simulink model "rti1401_program_nova"  (R2017b)
settings: Solver=ode1  StartTime=0.0  StopTime=Inf  FixedStep=0.001  RelTol=1e-3  EnableMultiTasking=on
PreLoadFcn:
  | dataCar
  | load_vars
  | structAero
  | structEstimPar
  | structSensors
  | structSettings
PostLoadFcn:
  | , if any(exist('dsrtsu_mdlpostloadfcn', 'file') == [2, 3, 6]), try dsrtsu_mdlpostloadfcn('Execute', bdroot); catch fprintf('Error in PostLoadFcn (dsrtsu_mdlpostloadfcn) for model "%s":\n %s\n', bdroot, lasterr); end, end,
InitFcn:
  | dataCar
  | load_vars
  | structAero
  | structEstimPar
  | structSensors
  | structSettings
StartFcn:
  | dataCar
  | load_vars
  | structAero
  | structEstimPar
  | structSensors
  | structSettings
values from neighbouring files (symbols this model uses):
  Throttle_limits = [0.15, 0.90, 0.16, 0.92]    [load_vars.m]
libraries: rtican x44, hdlsllib x32, simulink x8, rti1401lib_II_base x1, fuzblock x1
(part 3 of 11)

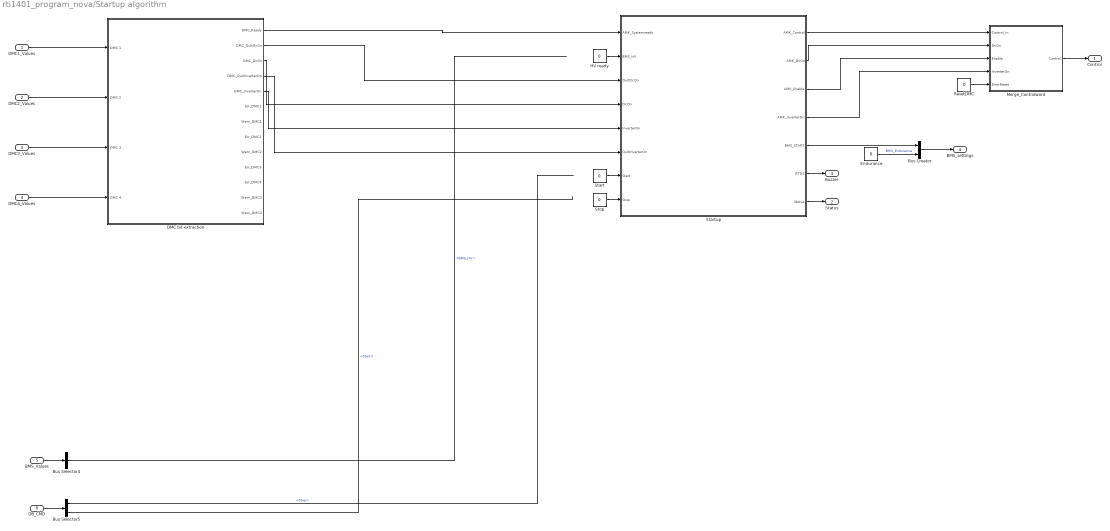
== system rti1401_program_nova/Startup algorithm ==
  DMC1_Values : Inport
  DMC2_Values : Inport  Port=2
  DMC3_Values : Inport  Port=3
  DMC4_Values : Inport  Port=4
  BMS_Values : Inport  Port=5
  DB_CMD : Inport  Port=6
  Bus Creator : BusCreator  Inputs=2
  Bus Selector4 : BusSelector  OutputSignals=BMS_HV
  Bus Selector5 : BusSelector  OutputSignals=Stop,Start
  DMC bit extraction : Subsystem
  Endurance : Constant  Value=0
  HV ready : Constant  Value=0
  Merge_Controlword : Subsystem
  ResetDMC : Constant  Value=0
  Start : Constant  Value=0
  Startup : Stateflow chart  TreatAsAtomicUnit=on
  Stop : Constant  Value=0
  Control : Outport
  Status : Outport  Port=2
  Buzzer : Outport  Port=3
  BMS_settings : Outport  Port=4
  wires:
  DB_CMD/1 -> Bus Selector5/1
  BMS_Values/1 -> Bus Selector4/1
  DMC1_Values/1 -> DMC bit extraction/1(DMC 1)
  DMC2_Values/1 -> DMC bit extraction/2(DMC 2)
  DMC3_Values/1 -> DMC bit extraction/3(DMC 3)
  DMC4_Values/1 -> DMC bit extraction/4(DMC 4)
  DMC bit extraction/1(DMC_Ready) -> Startup/1(AMK_Systemready)
  Bus Selector5/1 -> ?  "<Stop>"
  Bus Selector5/2 -> ?  "<Start>"
  Bus Selector4/1 -> ?  "<BMS_HV>"
  Startup/1(AMK_Control) -> Merge_Controlword/1(Control_in)
  Startup/2(AMK_DcOn) -> Merge_Controlword/2(DcOn)
  Startup/3(AMK_Enable) -> Merge_Controlword/3(Enable)
  Startup/4(AMK_InverterOn) -> Merge_Controlword/4(InverterOn)
  ResetDMC/1 -> Merge_Controlword/5(ErrorReset)
  Merge_Controlword/1(Control) -> Control/1
  Startup/7(Status) -> Status/1
  Startup/6(RTDS) -> Buzzer/1
  Startup/5(BMS_START) -> Bus Creator/1
  Endurance/1 -> Bus Creator/2  "BMS_Endurance"
  Bus Creator/1 -> BMS_settings/1
  HV ready/1 -> Startup/2(BMS_HV)
  DMC bit extraction/2(DMC_QuitDcOn) -> Startup/3(QuitDcOn)
  DMC bit extraction/3(DMC_DcOn) -> Startup/4(DcOn)
  DMC bit extraction/5(DMC_InverterOn) -> Startup/5(InverterOn)
  DMC bit extraction/4(DMC_QuitInverterOn) -> Startup/6(QuitInverterOn)
  Start/1 -> Startup/7(Start)
  Stop/1 -> Startup/8(Stop)

== system rti1401_program_nova/Inputs/Batpack ==
  Bus Creator : BusCreator  Inputs=19
  CAN_BMS_Values : rtican/RTICAN Receive (RX)   Reserved1=[]  Reserved2=[]  Reserved3=[]  Reserved4=[]  SfcnMessage=[]  Msg_Struct=[]  BoardTypeNo=[]  BoardNo=[]  ChannelNo=[]  Parameters=[]  DialogFcn=[]  UnitName=[]  Revision=[]  UnitValues=[]  DSProperties=struct('RTI',struct('Version',uint32(5),'BlockType',struct('isSLSource',uint8(1),'isSLSink',uint8(1),'isHWSource',uint8(0),'isHWSink',uint8(0),'isSetup',uint8(0),'isInline',uint8(1),'isNonInline',uint8(0),'isInterrupt',uint8(0),'isChannelwise',uint8(0)),'IOBoardType','RTICAN','UnitType','MESSAGE','Identifier','RX','DialogType','MSVC','BlockSet','RTICAN','SlaveProcessor','CAN'))  RTIBlockInterface=struct('OutputPortsWidth',int32([1 1 1 1 1 1 1 1 1 1 1 1 1 1 1 1 1 1 1]),'OutputPortsActive',[1 1 1 1 1 1 1 1 1 1 1 1 1 1 1 1 1 1 1],'OutputPortsName',{{'BMS_Total_Voltage','BMS_SoC','BMS_M1','BMS_M2','BMS_M3','BMS_M4','BMS_BOTS','BMS_Inertia','BMS_Interlock','BMS_BSPD','BMS_TSMS','BMS_IMD','BMS_Status','BMS_Voltage_Err','BMS_Temp_Err','BMS_HVD','BMS_Temp_Warn','BMS_Voltage_Warn','BMS_HV'}},'OutputPortsDataType',{{'SS_UINT16','SS_UINT16','SS_BOOLEAN','SS_BOOLEAN','SS_BOOLEAN','SS_BOOLEAN','SS_BOOLEAN','SS_BOOLEAN','SS_BOOLEAN','SS_BOOLEAN','SS_BOOLEAN','SS_BOOLEAN','SS_BOOLEAN','SS_BOOLEAN','SS_BOOLEAN','SS_BOOLEAN','SS_BOOLEAN','SS_BOOLEAN','SS_BOOLEAN'}},'OutputPortsLabel',{{'BMS_Total_Voltage','BMS_SoC','BMS_M1','BMS_M2','BMS_M3','BMS_M4','BMS_BOTS','BMS_Inertia','BMS_Interlock','BMS_BSPD','BMS_TSMS','BMS_IMD','BMS_Status','BMS_Voltage_Err','BMS_Temp_Err','BMS_HVD','BMS_Temp_Warn','BMS_Voltage_Warn','BMS_HV'}},'OutputPortsLabelMode','ON','InputPortsWidth',int32(0),'InputPortsActive',0,'DialogFcn','rtican_message_interface_gui','BlockDisplay',{{'','center'}},'IconTransparency','on','ParameterTunableNames',{{}},'InitLevel',3,'BlockName',struct('Token',{{'CAN_TYPE','_RX_M','_C'}},'BlockParam',{{'BoardTypeNo','BoardNo','ChannelNo'}}),'SampleTime',{{-1}},'TriggerPort',{{'none'}},'EnablePort',{{'none'}})  RTIBlockParameters=struct('BoardTypeNo',{{1,'OFF',[]}},'BoardNo',{{2,'ON',[1 16]}},'ChannelNo',{{2,'ON',[1 2]}},'Parameters',{{struct('DataFileSupport',struct('DataFileSelectedMaster',0,'DataFileSelectedLocal',0,'DataFileName',['<no datafile support>|'],'DataFileDate','','SelectedFile',['<no file selected>']),'Options',struct('StatusSelected',0,'TimeSelected',0,'DeltaTimeSelected',0,'BytePortSelected',0,'MessageLengthSelected',0,'TriggerPort',struct('Selected',0,'TriggerType',0),'UserCoding',struct('Selected',0,'InterfaceFile','UserDecodingFile','FcnName','UserDecodeFcn','InportSelected',0,'InportWidth',1,'OutportSelected',0,'OutportWidth',1),'EnablePortSelected',0,'SignalOnPortnameSelected',1,'UseRXService',0),'Message',struct('MsgOnBlocknameSelected',0,'MsgName','BMS_Values','MsgIdFormat',0,'MsgId',1,'MsgLength',7,'NumSignals',19,'SampleTime',-1,'Signal',struct('SgnName',{'BMS_Total_Voltage','BMS_SoC','BMS_M1','BMS_M2','BMS_M3','BMS_M4','BMS_BOTS','BMS_Inertia','BMS_Interlock','BMS_BSPD','BMS_TSMS','BMS_IMD','BMS_Status','BMS_Voltage_Err','BMS_Temp_Err','BMS_HVD','BMS_Temp_Warn','BMS_Voltage_Warn','BMS_HV'},'SgnStartBit',{0,16,32,33,34,35,36,37,38,39,40,41,42,43,44,45,46,47,48},'SgnLength',{16,16,1,1,1,1,1,1,1,1,1,1,1,1,1,1,1,1,1},'SgnType',{0,0,0,0,0,0,0,0,0,0,0,0,0,0,0,0,0,0,0},'ModeValue',{-1,-1,-1,-1,-1,-1,-1,-1,-1,-1,-1,-1,-1,-1,-1,-1,-1,-1,-1},'DataType',{0,0,0,0,0,0,0,0,0,0,0,0,0,0,0,0,0,0,0},'ByteLayout',{0,0,0,0,0,0,0,0,0,0,0,0,0,0,0,0,0,0,0},'Factor',{1,1,1,1,1,1,1,1,1,1,1,1,1,1,1,1,1,1,1},'Offset',{0,0,0,0,0,0,0,0,0,0,0,0,0,0,0,0,0,0,0},'SgnComment',{{''},{''},{''},{''},{''},{''},{''},{''},{''},{''},{''},{''},{''},{''},{''},{''},{''},{''},{''}},'SgnUnit',{'','','','','','','','','','','','','','','','','','',''},'Min',{0,0,0,0,0,0,0,0,0,0,0,0,0,0,0,0,0,0,0},'Max',{255,255,255,255,255,255,255,255,255,255,255,255,255,255,255,255,255,255,255},'SLDataType',{'SS_UINT16','SS_UINT16','SS_BOOLEAN','SS_BOOLEAN','SS_BOOLEAN','SS_BOOLEAN','SS_BOOLEAN','SS_BOOLEAN','SS_BOOLEAN','SS_BOOLEAN','SS_BOOLEAN','SS_BOOLEAN','SS_BOOLEAN','SS_BOOLEAN','SS_BOOLEAN','SS_BOOLEAN','SS_BOOLEAN','SS_BOOLEAN','SS_BOOLEAN'}),'MsgIdNumFormat',1,'MsgComment',{{''}}),'Version',1.2,'general',struct('isFromLib',0)),'OFF',[]}},'GroupId',{{struct('Group',{{'RTICAN'}},'No',4,'Behavior',{{'NAMECHANGE'}},'BlockType',{{'SINK'}},'NameChangeFlag',0),'OFF',[]}},'SFcnRTICANMessage',{{struct('MsgType','RX','SFcnPortType','Scalar','MsgName','BMS_Values','MsgIdFormat','STD','MsgId',1,'MsgLength',7,'NumSignals',19,'SampleTime',-1,'Signal',struct('SgnName',{'BMS_Total_Voltage','BMS_SoC','BMS_M1','BMS_M2','BMS_M3','BMS_M4','BMS_BOTS','BMS_Inertia','BMS_Interlock','BMS_BSPD','BMS_TSMS','BMS_IMD','BMS_Status','BMS_Voltage_Err','BMS_Temp_Err','BMS_HVD','BMS_Temp_Warn','BMS_Voltage_Warn','BMS_HV'},'SgnStartBit',{0,16,32,33,34,35,36,37,38,39,40,41,42,43,44,45,46,47,48},'SgnLength',{16,16,1,1,1,1,1,1,1,1,1,1,1,1,1,1,1,1,1},'SgnType',{'standard','standard','standard','standard','standard','standard','standard','standard','standard','standard','standard','standard','standard','standard','standard','standard','standard','standard','standard'},'ModeValue',{-1,-1,-1,-1,-1,-1,-1,-1,-1,-1,-1,-1,-1,-1,-1,-1,-1,-1,-1},'DataType',{['unsigned int'],['unsigned int'],['unsigned int'],['unsigned int'],['unsigned int'],['unsigned int'],['unsigned int'],['unsigned int'],['unsigned int'],['unsigned int'],['unsigned int'],['unsigned int'],['unsigned int'],['unsigned int'],['unsigned int'],['unsigned int'],['unsigned int'],['unsigned int'],['unsigned int']},'ByteLayout',{['little endian'],['little endian'],['little endian'],['little endian'],['little endian'],['little endian'],['little endian'],['little endian'],['little endian'],['little endian'],['little endian'],['little endian'],['little endian'],['little endian'],['little endian'],['little endian'],['little endian'],['little endian'],['little endian']},'Factor',{1,1,1,1,1,1,1,1,1,1,1,1,1,1,1,1,1,1,1},'Offset',{0,0,0,0,0,0,0,0,0,0,0,0,0,0,0,0,0,0,0},'SLDataType',{'SS_UINT16','SS_UINT16','SS_BOOLEAN','SS_BOOLEAN','SS_BOOLEAN','SS_BOOLEAN','SS_BOOLEAN','SS_BOOLEAN','SS_BOOLEAN','SS_BOOLEAN','SS_BOOLEAN','SS_BOOLEAN','SS_BOOLEAN','SS_BOOLEAN','SS_BOOLEAN','SS_BOOLEAN','SS_BOOLEAN','SS_BOOLEAN','SS_BOOLEAN'}),'StatusSelected','no','TimeSelected','no','DeltaTimeSelected','no','BytePortSelected','no','MessageLengthSelected','no','TriggerPort',struct('Selected','no','TriggerType',0),'UserCoding',struct('Selected','no','InterfaceFile','UserDecodingFile','FcnName','UserDecodeFcn','InportSelected','no','InportWidth',1,'OutportSelected','no','OutportWidth',1),'EnablePortSelected','no','UseRXService','no','BoardType','DS1','BoardNo',2,'ControllerNo',2),'OFF',[]}},'TLCFileName',{{'rtican_rx_message','OFF',[]}})  RTISFcnParameters=struct('SFcnRTICANMessage','struct','TLCFileName','char')  RTIBlockParaDefault=struct('BoardTypeNo',4302,'BoardNo',1,'ChannelNo',1,'Parameters',struct('DataFileSupport',struct('DataFileSelectedMaster',0,'DataFileSelectedLocal',0,'DataFileName','','DataFileDate','','SelectedFile',['<no file selected>']),'Options',struct('StatusSelected',1,'TimeSelected',1,'DeltaTimeSelected',1,'BytePortSelected',0,'MessageLengthSelected',0,'TriggerPort',struct('Selected',0,'TriggerType','rising'),'UserCoding',struct('Selected',0,'InterfaceFile','UserDecodingFile','FcnName','UserDecodeFcn','InportSelected',0,'InportWidth',1,'OutportSelected',0,'OutportWidth',1),'EnablePortSelected',0,'SignalOnPortnameSelected',1,'UseRXService',0),'Message',struct('MsgOnBlocknameSelected',0,'MsgName',['RX Message'],'MsgIdFormat',0,'MsgId',100,'MsgLength',8,'NumSignals',1,'SampleTime',-1,'Signal',struct('SgnName',['RX signal'],'SgnStartBit',0,'SgnLength',8,'SgnType',0,'ModeValue',-1,'DataType',0,'SLDataType','SS_DOUBLE','ByteLayout',0,'Factor',1,'Offset',0,'Min',0,'Max',255,'SgnComment',{{}},'SgnUnit',''),'MsgIdNumFormat',0,'MsgComment',{{''}}),'Version',1.2,'general',struct('isFromLib',1)),'GroupId',struct('Group',{{'RTICAN'}},'No',1,'Behavior',{{'NAMECHANGE'}},'BlockType',{{'SINK'}},'NameChangeFlag',0),'SFcnRTICANMessage',struct('MsgType','RX','MsgName',['RX Message'],'MsgIdFormat','STD','MsgId',100,'MsgLength',8,'NumSignals',1,'SampleTime',-1,'Signal',struct('SgnName',['RX signal'],'SgnStartBit',0,'SgnLength',8,'SgnType','standard','ModeValue',-1,'DataType',['unsigned int'],'ByteLayout',['little endian'],'SLDataType','SS_DOUBLE','Factor',1,'Offset',0),'StatusSelected','yes','TimeSelected','yes','DeltaTimeSelected','yes','BytePortSelected','no','MessageLengthSelected','no','EnablePortSelected','no','UserCoding',struct('Selected','no','InterfaceFile','UserDecodingFile','FcnName','UserDecodeFcn','InportSelected','no','InportWidth',1,'OutportSelected','no','OutportWidth',1),'TriggerPort',struct('Selected','no','TriggerType','rising'),'UseRXService','no','BoardType','DS4302','BoardNo',1,'ControllerNo',1,'SFcnPortType','Scalar'),'TLCFileName','rtican_rx_message')
      settings: AttributesFormatString=Group Id: RTICAN4\n
  BMS_Values : Outport
  wires:
  CAN_BMS_Values/19 -> Bus Creator/19  "BMS_HV"
  CAN_BMS_Values/18 -> Bus Creator/18  "BMS_Voltage_Warn"
  CAN_BMS_Values/17 -> Bus Creator/17  "BMS_Temp_Warn"
  CAN_BMS_Values/16 -> Bus Creator/16  "BMS_HVD"
  CAN_BMS_Values/15 -> Bus Creator/15  "BMS_Temp_Err"
  CAN_BMS_Values/14 -> Bus Creator/14  "BMS_Voltage_Err"
  CAN_BMS_Values/13 -> Bus Creator/13  "BMS_Status"
  CAN_BMS_Values/12 -> Bus Creator/12  "BMS_IMD"
  CAN_BMS_Values/11 -> Bus Creator/11  "BMS_TSMS"
  CAN_BMS_Values/10 -> Bus Creator/10  "BMS_BSPD"
  CAN_BMS_Values/9 -> Bus Creator/9  "BMS_Interlock"
  CAN_BMS_Values/8 -> Bus Creator/8  "BMS_Inertia"
  CAN_BMS_Values/7 -> Bus Creator/7  "BMS_BOTS"
  CAN_BMS_Values/6 -> Bus Creator/6  "BMS_M4"
  CAN_BMS_Values/5 -> Bus Creator/5  "BMS_M3"
  CAN_BMS_Values/4 -> Bus Creator/4  "BMS_M2"
  CAN_BMS_Values/3 -> Bus Creator/3  "BMS_M1"
  CAN_BMS_Values/2 -> Bus Creator/2  "BMS_SoC"
  CAN_BMS_Values/1 -> Bus Creator/1  "BMS_Total_Voltage"
  Bus Creator/1 -> BMS_Values/1

== system rti1401_program_nova/Inputs/Commands ==
  Bus Creator : BusCreator  Inputs=10
  CAN_TYPE1_RX_M1_C1 : rtican/RTICAN Receive (RX)   Reserved1=[]  Reserved2=[]  Reserved3=[]  Reserved4=[]  SfcnMessage=[]  Msg_Struct=[]  BoardTypeNo=[]  BoardNo=[]  ChannelNo=[]  Parameters=[]  DialogFcn=[]  UnitName=[]  Revision=[]  UnitValues=[]  DSProperties=struct('RTI',struct('Version',uint32(5),'BlockType',struct('isSLSource',uint8(1),'isSLSink',uint8(1),'isHWSource',uint8(0),'isHWSink',uint8(0),'isSetup',uint8(0),'isInline',uint8(1),'isNonInline',uint8(0),'isInterrupt',uint8(0),'isChannelwise',uint8(0)),'IOBoardType','RTICAN','UnitType','MESSAGE','Identifier','RX','DialogType','MSVC','BlockSet','RTICAN','SlaveProcessor','CAN'))  RTIBlockInterface=struct('OutputPortsWidth',int32([1 1 1 1 1 1 1 1 1]),'OutputPortsActive',[1 1 1 1 1 1 1 1 1],'OutputPortsName',{{'Start','Stop','TV','Power','MxFz','Regen','Traction','FxInf','YRC'}},'OutputPortsDataType',{{'SS_BOOLEAN','SS_BOOLEAN','SS_UINT8','SS_UINT8','SS_UINT8','SS_UINT8','SS_BOOLEAN','SS_BOOLEAN','SS_BOOLEAN'}},'OutputPortsLabel',{{'Start','Stop','TV','Power','MxFz','Regen','Traction','FxInf','YRC'}},'OutputPortsLabelMode','ON','InputPortsWidth',int32(0),'InputPortsActive',0,'DialogFcn','rtican_message_interface_gui','BlockDisplay',{{'','center'}},'IconTransparency','on','ParameterTunableNames',{{}},'InitLevel',3,'BlockName',struct('Token',{{'CAN_TYPE','_RX_M','_C'}},'BlockParam',{{'BoardTypeNo','BoardNo','ChannelNo'}}),'SampleTime',{{-1}},'TriggerPort',{{'none'}},'EnablePort',{{'none'}})  RTIBlockParameters=struct('BoardTypeNo',{{1,'OFF',[]}},'BoardNo',{{1,'ON',[1 16]}},'ChannelNo',{{1,'ON',[1 2]}},'Parameters',{{struct('DataFileSupport',struct('DataFileSelectedMaster',0,'DataFileSelectedLocal',0,'DataFileName',['<no datafile support>|'],'DataFileDate','','SelectedFile',['<no file selected>']),'Options',struct('StatusSelected',0,'TimeSelected',0,'DeltaTimeSelected',0,'BytePortSelected',0,'MessageLengthSelected',0,'TriggerPort',struct('Selected',0,'TriggerType',0),'UserCoding',struct('Selected',0,'InterfaceFile','UserDecodingFile','FcnName','UserDecodeFcn','InportSelected',0,'InportWidth',1,'OutportSelected',0,'OutportWidth',1),'EnablePortSelected',0,'SignalOnPortnameSelected',1,'UseRXService',0),'Message',struct('MsgOnBlocknameSelected',0,'MsgName','DB_CTRL','MsgIdFormat',0,'MsgId',17,'MsgLength',3,'NumSignals',9,'SampleTime',-1,'Signal',struct('SgnName',{'Start','Stop','TV','Power','MxFz','Regen','Traction','FxInf','YRC'},'SgnStartBit',{0,1,2,4,8,16,20,21,22},'SgnLength',{1,1,2,4,8,4,1,1,1},'SgnType',{0,0,0,0,0,0,0,0,0},'ModeValue',{-1,-1,-1,-1,-1,-1,-1,-1,-1},'DataType',{0,0,0,0,0,0,0,0,0},'ByteLayout',{1,1,1,1,1,1,1,1,1},'Factor',{1,1,1,1,1,1,1,1,1},'Offset',{0,0,0,0,0,0,0,0,0},'SgnComment',{{''},{''},{''},{''},{''},{''},{''},{''},{''}},'SgnUnit',{'','','','','','','','',''},'Min',{0,0,0,0,0,0,0,0,0},'Max',{255,255,255,255,255,255,255,255,255},'SLDataType',{'SS_BOOLEAN','SS_BOOLEAN','SS_UINT8','SS_UINT8','SS_UINT8','SS_UINT8','SS_BOOLEAN','SS_BOOLEAN','SS_BOOLEAN'}),'MsgIdNumFormat',1,'MsgComment',{{''}}),'Version',1.2,'general',struct('isFromLib',0)),'OFF',[]}},'GroupId',{{struct('Group',{{'RTICAN'}},'No',1,'Behavior',{{'NAMECHANGE'}},'BlockType',{{'SINK'}},'NameChangeFlag',0),'OFF',[]}},'SFcnRTICANMessage',{{struct('MsgType','RX','SFcnPortType','Scalar','MsgName','DB_CTRL','MsgIdFormat','STD','MsgId',17,'MsgLength',3,'NumSignals',9,'SampleTime',-1,'Signal',struct('SgnName',{'Start','Stop','TV','Power','MxFz','Regen','Traction','FxInf','YRC'},'SgnStartBit',{0,1,2,4,8,16,20,21,22},'SgnLength',{1,1,2,4,8,4,1,1,1},'SgnType',{'standard','standard','standard','standard','standard','standard','standard','standard','standard'},'ModeValue',{-1,-1,-1,-1,-1,-1,-1,-1,-1},'DataType',{['unsigned int'],['unsigned int'],['unsigned int'],['unsigned int'],['unsigned int'],['unsigned int'],['unsigned int'],['unsigned int'],['unsigned int']},'ByteLayout',{['big endian'],['big endian'],['big endian'],['big endian'],['big endian'],['big endian'],['big endian'],['big endian'],['big endian']},'Factor',{1,1,1,1,1,1,1,1,1},'Offset',{0,0,0,0,0,0,0,0,0},'SLDataType',{'SS_BOOLEAN','SS_BOOLEAN','SS_UINT8','SS_UINT8','SS_UINT8','SS_UINT8','SS_BOOLEAN','SS_BOOLEAN','SS_BOOLEAN'}),'StatusSelected','no','TimeSelected','no','DeltaTimeSelected','no','BytePortSelected','no','MessageLengthSelected','no','TriggerPort',struct('Selected','no','TriggerType',0),'UserCoding',struct('Selected','no','InterfaceFile','UserDecodingFile','FcnName','UserDecodeFcn','InportSelected','no','InportWidth',1,'OutportSelected','no','OutportWidth',1),'EnablePortSelected','no','UseRXService','no','BoardType','DS1','BoardNo',1,'ControllerNo',1),'OFF',[]}},'TLCFileName',{{'rtican_rx_message','OFF',[]}})  RTISFcnParameters=struct('SFcnRTICANMessage','struct','TLCFileName','char')  RTIBlockParaDefault=struct('BoardTypeNo',4302,'BoardNo',1,'ChannelNo',1,'Parameters',struct('DataFileSupport',struct('DataFileSelectedMaster',0,'DataFileSelectedLocal',0,'DataFileName','','DataFileDate','','SelectedFile',['<no file selected>']),'Options',struct('StatusSelected',1,'TimeSelected',1,'DeltaTimeSelected',1,'BytePortSelected',0,'MessageLengthSelected',0,'TriggerPort',struct('Selected',0,'TriggerType','rising'),'UserCoding',struct('Selected',0,'InterfaceFile','UserDecodingFile','FcnName','UserDecodeFcn','InportSelected',0,'InportWidth',1,'OutportSelected',0,'OutportWidth',1),'EnablePortSelected',0,'SignalOnPortnameSelected',1,'UseRXService',0),'Message',struct('MsgOnBlocknameSelected',0,'MsgName',['RX Message'],'MsgIdFormat',0,'MsgId',100,'MsgLength',8,'NumSignals',1,'SampleTime',-1,'Signal',struct('SgnName',['RX signal'],'SgnStartBit',0,'SgnLength',8,'SgnType',0,'ModeValue',-1,'DataType',0,'SLDataType','SS_DOUBLE','ByteLayout',0,'Factor',1,'Offset',0,'Min',0,'Max',255,'SgnComment',{{}},'SgnUnit',''),'MsgIdNumFormat',0,'MsgComment',{{''}}),'Version',1.2,'general',struct('isFromLib',1)),'GroupId',struct('Group',{{'RTICAN'}},'No',1,'Behavior',{{'NAMECHANGE'}},'BlockType',{{'SINK'}},'NameChangeFlag',0),'SFcnRTICANMessage',struct('MsgType','RX','MsgName',['RX Message'],'MsgIdFormat','STD','MsgId',100,'MsgLength',8,'NumSignals',1,'SampleTime',-1,'Signal',struct('SgnName',['RX signal'],'SgnStartBit',0,'SgnLength',8,'SgnType','standard','ModeValue',-1,'DataType',['unsigned int'],'ByteLayout',['little endian'],'SLDataType','SS_DOUBLE','Factor',1,'Offset',0),'StatusSelected','yes','TimeSelected','yes','DeltaTimeSelected','yes','BytePortSelected','no','MessageLengthSelected','no','EnablePortSelected','no','UserCoding',struct('Selected','no','InterfaceFile','UserDecodingFile','FcnName','UserDecodeFcn','InportSelected','no','InportWidth',1,'OutportSelected','no','OutportWidth',1),'TriggerPort',struct('Selected','no','TriggerType','rising'),'UseRXService','no','BoardType','DS4302','BoardNo',1,'ControllerNo',1,'SFcnPortType','Scalar'),'TLCFileName','rtican_rx_message')
      settings: AttributesFormatString=Group Id: RTICAN1\n
  Constant{,1..3} (4 alike) : Constant  Value=0
  Power : Constant  Value=0  OutDataTypeStr=uint8
  TV : Constant  Value=0  OutDataTypeStr=uint8
  Dash_Commands : Outport
  wires:
  CAN_TYPE1_RX_M1_C1/1 -> Bus Creator/5  "Start"
  CAN_TYPE1_RX_M1_C1/2 -> Bus Creator/6  "Stop"
  CAN_TYPE1_RX_M1_C1/5 -> Bus Creator/9  "MxFz"
  CAN_TYPE1_RX_M1_C1/6 -> Bus Creator/10  "Regen"
  Bus Creator/1 -> Dash_Commands/1
  Constant/1 -> Bus Creator/1  "effEstimation"
  Constant1/1 -> Bus Creator/2  "unlimitedFx"
  Constant2/1 -> Bus Creator/3  "TC"
  Constant3/1 -> Bus Creator/4  "YRC"
  TV/1 -> Bus Creator/7  "TV"
  Power/1 -> Bus Creator/8  "Power"
